simulink model "ModelEquationsDOF3"  (R2022b)
settings: Solver=ode4  StartTime=0.0  StopTime=100  FixedStep=10^-3  RelTol=1e-3
values from neighbouring files (symbols this model uses):
  Cc = 900    [ModelFixedParamDOF3.m]
  Cs = 74518    [OptimizedParamDOF3.m]    (also in OptimizedParamDOF4.m = 900)
  Ct = 850    [ModelFixedParamDOF3.m]    (also in ModelFixedParamDOF4.m)
  Kc = 10039    [ModelFixedParamDOF3.m]
  Ks = 106826    [OptimizedParamDOF3.m]    (also in OptimizedParamDOF4.m = 10039)
  Kt = 150000    [ModelFixedParamDOF3.m]    (also in ModelFixedParamDOF4.m)
  mc = 441    [ModelFixedParamDOF3.m]    (also in ModelFixedParamDOF5.m = 75)
  ms = 237    [ModelFixedParamDOF2.m]    (also in ModelFixedParamDOF3.m = 35; ModelFixedParamDOF5.m = 730)
  mt = 25    [ModelFixedParamDOF3.m]
  road_front_wheel = M.'    [LoadRoadScript.m]
settings Model: Creator=Ade  LastModifiedBy=andre
settings SolverCC: AlgebraicLoopSolver=TrustRegion
settings DataIOCC: ReturnWorkspaceOutputs=off
settings DebuggingCC: UnconnectedInputMsg=warning  UnconnectedOutputMsg=warning  UnconnectedLineMsg=warning  SFMachineParentedDataDiag=warning  ArithmeticOperatorsInVariantConditions=warning
settings ModelReferenceCC: EnableRefExpFcnMdlSchedulingChecks=on
settings SFSimCC: SimUseLocalCustomCode=off  CustomCodeUndefinedFunction=UseInterfaceOnly
settings RTWCC: RTWUseLocalCustomCode=off  DLArmComputeVersion=19.05

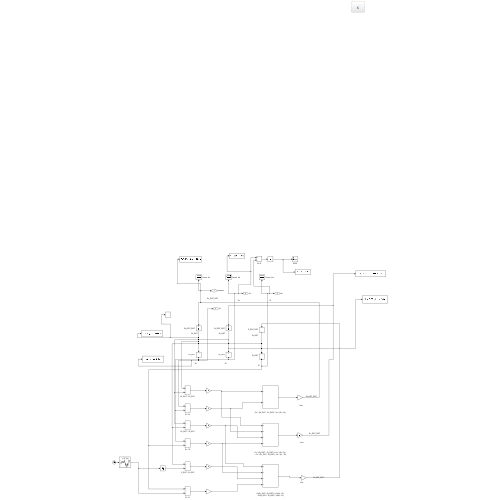
[thumbnail: Simulink's stored preview of the top-level diagram]
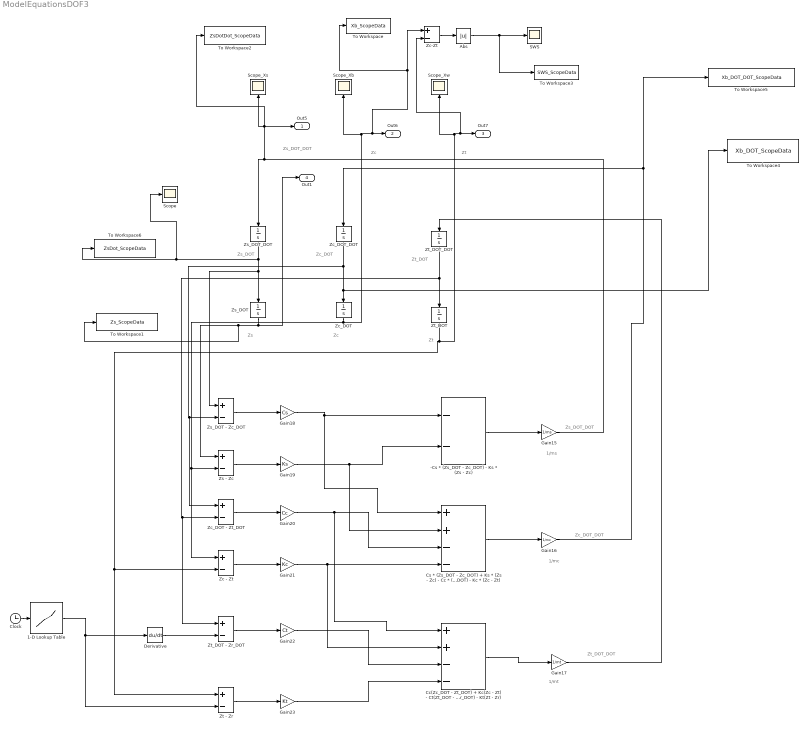
== system ModelEquationsDOF3 ==
  note: 1/mt
  note: Zs_DOT
  note: Zs
  note: Zc
  note: Zc_DOT
  note: Zt
  note: Zt_DOT
  note: Zs_DOT_DOT
  note: Zt_DOT_DOT
  note: Zc_DOT_DOT
  note: 1/mc
  note: 1/ms
  note: Zs_DOT_DOT
  note: Zc
  note: Zt
  " Cc(Zc_DOT - Zt_DOT) + Kc(Zc - Zt) - Ct(Zt_DOT - Zr_DOT) - Kt(Zt - Zr)" : Sum  Inputs=++--
  " Cs * (Zs_DOT - Zc_DOT) + Ks * (Zs - Zc) - Cc * (Zc_DOT - Zt_DOT) - Kc * (Zc - Zt)" : Sum  Inputs=++--
  " -Cs * (Zs_DOT - Zc_DOT) - Ks * (Zs - Zc) " : Sum  Inputs=--
  1-D Lookup Table : Lookup_n-D  NumberOfTableDimensions=1  LookupTableObject=road_front_wheel  BreakpointsForDimension1=[1:100]  Table=road_front_wheel  InternalRulePriority=Speed  RndMeth=Simplest
  Abs : Abs  SaturateOnIntegerOverflow=off
  Clock : Clock
  Derivative : Derivative
  Gain15 : Gain  Gain=1/ms
  Gain16 : Gain  Gain=1/mc
  Gain17 : Gain  Gain=1/mt
  Gain18 : Gain  Gain=Cs
  Gain19 : Gain  Gain=Ks
  Gain20 : Gain  Gain=Cc
  Gain21 : Gain  Gain=Kc
  Gain22 : Gain  Gain=Ct
  Gain23 : Gain  Gain=Kt
  SWS : Scope
  Scope : Scope
  Scope_Xb : Scope
  Scope_Xs : Scope
  Scope_Xw : Scope
  To Workspace : ToWorkspace  VariableName=Xb_ScopeData  SaveFormat=Structure With Time  SampleTime=-1
  To Workspace1 : ToWorkspace  VariableName=Zs_ScopeData  SaveFormat=Structure With Time  SampleTime=-1
  To Workspace2 : ToWorkspace  VariableName=ZsDotDot_ScopeData  SaveFormat=Structure With Time  SampleTime=-1
  To Workspace3 : ToWorkspace  VariableName=SWS_ScopeData  SaveFormat=Structure With Time  SampleTime=-1
  To Workspace4 : ToWorkspace  VariableName=Xb_DOT_ScopeData  SaveFormat=Structure With Time  SampleTime=-1
  To Workspace5 : ToWorkspace  VariableName=Xb_DOT_DOT_ScopeData  SaveFormat=Structure With Time  SampleTime=-1
  To Workspace6 : ToWorkspace  VariableName=ZsDot_ScopeData  SaveFormat=Structure With Time  SampleTime=-1
  Zc - Zt : Sum  Inputs=+-
  Zc-Zt : Sum  Inputs=+-
  Zc_DOT : Integrator
  Zc_DOT - Zt_DOT : Sum  Inputs=+-
  Zc_DOT_DOT : Integrator
  Zs - Zc : Sum  Inputs=+-
  Zs_DOT : Integrator
  Zs_DOT - Zc_DOT : Sum  Inputs=+-
  Zs_DOT_DOT : Integrator
  Zt - Zr : Sum  Inputs=+-
  "Zt_DOT " : Integrator
  "Zt_DOT - Zr_DOT " : Sum  Inputs=+-
  "Zt_DOT_DOT " : Integrator
  Out5 : Outport  SignalName=ZsDotDot  VectorParamsAs1DForOutWhenUnconnected=off
  Out6 : Outport  Port=2  SignalName=Xb  VectorParamsAs1DForOutWhenUnconnected=off
  Out7 : Outport  Port=3  SignalName=Xw  VectorParamsAs1DForOutWhenUnconnected=off
  Out1 : Outport  Port=4  SignalName=Zs
  wires:
  Zs_DOT_DOT/1 -> Scope/1, To Workspace6/1, Zs_DOT - Zc_DOT/1, Zs_DOT/1
  Zs_DOT/1 -> Out1/1, To Workspace1/1, Zs - Zc/1
  Zc_DOT/1 -> Scope_Xb/1, To Workspace/1, Zc-Zt/1, Out6/1, Zc - Zt/1, Zs - Zc/2
  Zc_DOT_DOT/1 -> Zc_DOT - Zt_DOT/1, Zs_DOT - Zc_DOT/2, Zc_DOT/1, To Workspace4/1
  " -Cs * (Zs_DOT - Zc_DOT) - Ks * (Zs - Zc) "/1 -> Gain15/1
  " Cs * (Zs_DOT - Zc_DOT) + Ks * (Zs - Zc) - Cc * (Zc_DOT - Zt_DOT) - Kc * (Zc - Zt)"/1 -> Gain16/1
  " Cc(Zc_DOT - Zt_DOT) + Kc(Zc - Zt) - Ct(Zt_DOT - Zr_DOT) - Kt(Zt - Zr)"/1 -> Gain17/1
  Zs - Zc/1 -> Gain19/1
  Zs_DOT - Zc_DOT/1 -> Gain18/1
  Zc - Zt/1 -> Gain21/1
  Zc_DOT - Zt_DOT/1 -> Gain20/1
  Zt - Zr/1 -> Gain23/1
  "Zt_DOT - Zr_DOT "/1 -> Gain22/1
  Gain23/1 -> " Cc(Zc_DOT - Zt_DOT) + Kc(Zc - Zt) - Ct(Zt_DOT - Zr_DOT) - Kt(Zt - Zr)"/4
  Gain22/1 -> " Cc(Zc_DOT - Zt_DOT) + Kc(Zc - Zt) - Ct(Zt_DOT - Zr_DOT) - Kt(Zt - Zr)"/3
  Gain21/1 -> " Cc(Zc_DOT - Zt_DOT) + Kc(Zc - Zt) - Ct(Zt_DOT - Zr_DOT) - Kt(Zt - Zr)"/2, " Cs * (Zs_DOT - Zc_DOT) + Ks * (Zs - Zc) - Cc * (Zc_DOT - Zt_DOT) - Kc * (Zc - Zt)"/4
  Gain20/1 -> " Cc(Zc_DOT - Zt_DOT) + Kc(Zc - Zt) - Ct(Zt_DOT - Zr_DOT) - Kt(Zt - Zr)"/1, " Cs * (Zs_DOT - Zc_DOT) + Ks * (Zs - Zc) - Cc * (Zc_DOT - Zt_DOT) - Kc * (Zc - Zt)"/3
  Gain18/1 -> " -Cs * (Zs_DOT - Zc_DOT) - Ks * (Zs - Zc) "/1, " Cs * (Zs_DOT - Zc_DOT) + Ks * (Zs - Zc) - Cc * (Zc_DOT - Zt_DOT) - Kc * (Zc - Zt)"/1
  Gain19/1 -> " -Cs * (Zs_DOT - Zc_DOT) - Ks * (Zs - Zc) "/2, " Cs * (Zs_DOT - Zc_DOT) + Ks * (Zs - Zc) - Cc * (Zc_DOT - Zt_DOT) - Kc * (Zc - Zt)"/2
  "Zt_DOT_DOT "/1 -> "Zt_DOT - Zr_DOT "/1, Zc_DOT - Zt_DOT/2, "Zt_DOT "/1
  Gain16/1 -> To Workspace5/1, Zc_DOT_DOT/1
  Gain17/1 -> "Zt_DOT_DOT "/1
  1-D Lookup Table/1 -> Derivative/1, Zt - Zr/2
  "Zt_DOT "/1 -> Scope_Xw/1, Zc-Zt/2, Out7/1, Zt - Zr/1, Zc - Zt/2
  Zc-Zt/1 -> Abs/1
  Gain15/1 -> To Workspace2/1, Scope_Xs/1, Out5/1, Zs_DOT_DOT/1
  Clock/1 -> 1-D Lookup Table/1
  Abs/1 -> To Workspace3/1, SWS/1
  Derivative/1 -> "Zt_DOT - Zr_DOT "/2
